simulink model "R7014E_DoubleTankSim2018a"  (R2018a)
settings: Solver=ode5  StartTime=0.0  StopTime=500  RelTol=1e-3  EnableMultiTasking=on
values from neighbouring files (symbols this model uses):
  A = A_const * [-1/sqrt(2*g*(h1+h_eq)) 0 ... (first row only)    [myTank.m]
  B = [6.95/36.2; 0]    [myTank.m]
  C = [0 1]    [myTank.m]
  K = (P*C' + N*R)*inv(R)    [myTank.m]
Description:
  | Double tank process simulation model
  | V1.0
  | 
  | Author: Wolfgang Birk, LTU
settings Model: MinMaxOverflowLogging=ForceOff  Creator=wolfgang  LastModifiedBy=oskwij-4
settings DataIOCC: LimitDataPoints=on  SaveFormat=Array  SignalLoggingSaveFormat=ModelDataLogs
settings OptimizationCC: ExpressionDepthLimit=2147483647  LifeSpan=inf
settings DebuggingCC: UnderspecifiedInitializationDetection=Classic  MergeDetectMultiDrivingBlocksExec=none  SolverPrmCheckMsg=warning  FcnCallInpInsideContextMsg=warning  StateNameClashWarn=warning  SFUnexpectedBacktrackingDiag=warning  SFNoUnconditionalDefaultTransitionDiag=warning  SFExecutionAtInitializationDiag=none
settings HardwareCC: ProdBitPerPointer=32  ProdBitPerSizeT=32  ProdBitPerPtrDiffT=32  ProdLargestAtomicFloat=None  ProdIntDivRoundTo=Undefined  ProdEndianess=Unspecified  ProdWordSize=32  ProdHWDeviceType=32-bit Generic
settings ModelReferenceCC: PropagateSignalLabelsOutOfModel=off
settings CodeAppCC: StateflowObjectComments=on
settings GRTTargetCC: TargetLangStandard=C89/C90 (ANSI)  GeneratePreprocessorConditionals=Disable all
settings ConfigComp: CovMetricSettings=dw  CovHtmlReporting=on  CovSaveCumulativeToWorkspaceVar=on  CovSaveSingleToWorkspaceVar=on  CovExternalEMLEnable=off

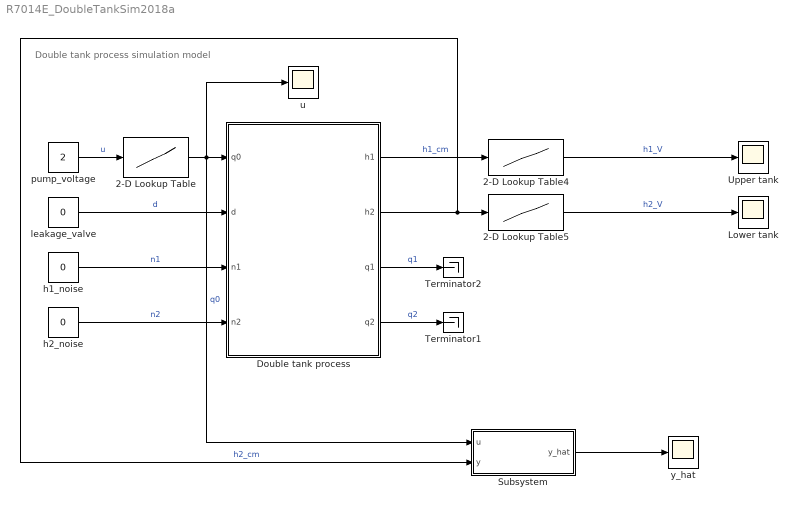
== system R7014E_DoubleTankSim2018a ==
  note: Double tank process simulation model
  2-D Lookup Table : Lookup_n-D  NumberOfTableDimensions=1  BreakpointsForDimension1=x  BreakpointsForDimension2=[1:3]  Table=y  RndMeth=Simplest  InputSameDT=on  mask{x=[0,1,2,3,4,5,6,7,8,9,10], y=|}
      mask y=|
      | [0.0,
      | 0.0,
      | 20.2,
      | 31.9,
      | 40.4,
      | 45.2,
      | 48.7,
      | 52.3,
      | 55.3,
      | 58.5,
      | 63.8]
      mask prompts: x "Values on x-axis"; y "Values on y-axis"
  2-D Lookup Table4 : Lookup_n-D  NumberOfTableDimensions=1  BreakpointsForDimension1=x  BreakpointsForDimension2=[1:3]  Table=y  RndMeth=Simplest  InputSameDT=on  mask{x=[2.50,3.00,3.50,4.00,4.50,5.00,5.50,6.00,6.50,7.00,7.50,8.00,8.50,9.00,9.50,10.00,10.50,11.00,11.50,12.00,12.50,13.00,13.50,14.00,14.50,15.00,15.50], y=[0.21,0.62,1.00,1.49,1.80,2.12,2.54,2.97,3.32,3.71,4.09,4.51,4.87,5.25,5.57,6.04,6.41,6.78,7.13,7.56,7.91,8.32,8.69,9.07,9.42,9.82,9.99]}
      mask prompts: x "Values on x-axis"; y "Values on y-axis"
  2-D Lookup Table5 : Lookup_n-D  NumberOfTableDimensions=1  BreakpointsForDimension1=x  BreakpointsForDimension2=[1:3]  Table=y  RndMeth=Simplest  InputSameDT=on  mask{x=[2.50,3.00,3.50,4.00,4.50,5.00,5.50,6.00,6.50,7.00,7.50,8.00,8.50,9.00,9.50,10.00,10.50,11.00,11.50,12.00,12.50,13.00,13.50,14.00,14.50,15.00,15.50], y=[0.10,0.47,0.87,1.23,1.57,1.98,2.41,2.77,3.16,3.53,3.94,4.32,4.71,5.10,5.46, 5.85, 6.24, 6.63, 7.02, 7.42, 7.74, 8.15, 8.52, 8.90, 9.28, 9.67, 9.94]}
      mask prompts: x "Values on x-axis"; y "Values on y-axis"
  Double tank process : Subsystem  mask{At=33, Ao=0.17, hmax=15.5}
      mask prompts: At "Tank area (cm^2)"; Ao "Opening area (cm^2)"; hmax "Tank height (cm)"
      mask help: Double tank process parameters
  Lower tank : Scope
  Subsystem : Subsystem
  Terminator1 : Terminator
  Terminator2 : Terminator
  Upper tank : Scope
  h1_noise : Constant  Value=0
  h2_noise : Constant  Value=0
  leakage_valve : Constant  Value=0
  pump_voltage : Constant  Value=2
  "u " : Scope
  "y_hat " : Scope
  wires:
  2-D Lookup Table4/1 -> Upper tank/1  "h1_V"
  leakage_valve/1 -> Double tank process/2(d)  "d"
  pump_voltage/1 -> 2-D Lookup Table/1  "u"
  2-D Lookup Table/1 -> Subsystem/1(u), "u "/1, Double tank process/1(q0)  "q0"
  Double tank process/1(h1) -> 2-D Lookup Table4/1  "h1_cm"
  Double tank process/2(h2) -> Subsystem/2(y), 2-D Lookup Table5/1  "h2_cm"
  Double tank process/4(q2) -> Terminator1/1  "q2"
  2-D Lookup Table5/1 -> Lower tank/1  "h2_V"
  Double tank process/3(q1) -> Terminator2/1  "q1"
  h1_noise/1 -> Double tank process/3(n1)  "n1"
  h2_noise/1 -> Double tank process/4(n2)  "n2"
  Subsystem/1("y_hat ") -> "y_hat "/1

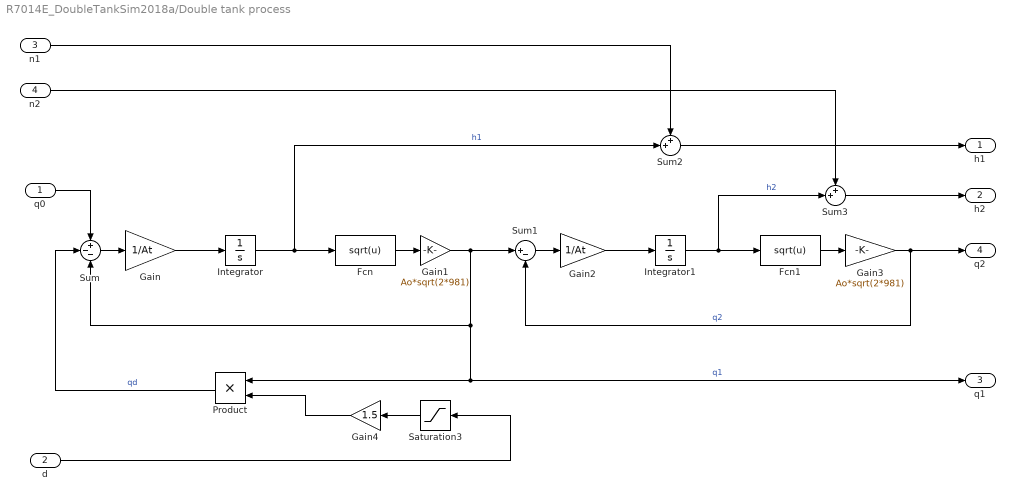
== system R7014E_DoubleTankSim2018a/Double tank process ==
  q0 : Inport
  d : Inport  Port=2
  n1 : Inport  Port=3
  n2 : Inport  Port=4
  Fcn : Fcn  Expr=sqrt(u)
  Fcn1 : Fcn  Expr=sqrt(u)
  Gain : Gain  Gain=1/At
  Gain1 : Gain  Gain=Ao*sqrt(2*981)
  Gain2 : Gain  Gain=1/At
  Gain3 : Gain  Gain=Ao*sqrt(2*981)
  Gain4 : Gain  Gain=1.5
  Integrator : Integrator  LimitOutput=on  UpperSaturationLimit=hmax  LowerSaturationLimit=0
  Integrator1 : Integrator  LimitOutput=on  UpperSaturationLimit=hmax  LowerSaturationLimit=0
  Product : Product  RndMeth=Zero
  Saturation3 : Saturate  UpperLimit=1  LowerLimit=0
  Sum : Sum  Inputs=+--
  Sum1 : Sum  Inputs=|+-
  Sum2 : Sum  Inputs=++|
  Sum3 : Sum  Inputs=++|
  h1 : Outport
  h2 : Outport  Port=2
  q1 : Outport  Port=3
  q2 : Outport  Port=4
  wires:
  Sum/1 -> Gain/1
  Gain/1 -> Integrator/1
  Fcn/1 -> Gain1/1
  Gain1/1 -> Sum1/1, Product/1, q1/1, Sum/3  "q1"
  Sum1/1 -> Gain2/1
  Gain2/1 -> Integrator1/1
  Fcn1/1 -> Gain3/1
  Gain3/1 -> Sum1/2, q2/1  "q2"
  q0/1 -> Sum/1
  Integrator/1 -> Sum2/2, Fcn/1  "h1"
  Product/1 -> Sum/2  "qd"
  d/1 -> Saturation3/1
  Integrator1/1 -> Sum3/2, Fcn1/1  "h2"
  Saturation3/1 -> Gain4/1
  Gain4/1 -> Product/2
  Sum2/1 -> h1/1
  n1/1 -> Sum2/1
  Sum3/1 -> h2/1
  n2/1 -> Sum3/1

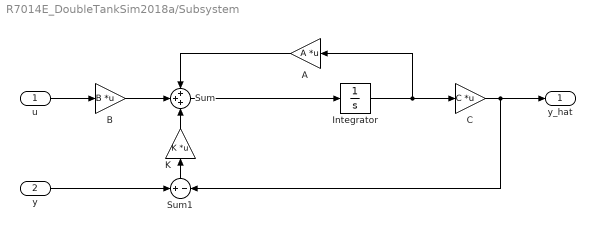
== system R7014E_DoubleTankSim2018a/Subsystem ==
  u : Inport
  y : Inport  Port=2
  A : Gain  Gain=A  Multiplication=Matrix(K*u)
  B : Gain  Gain=B  Multiplication=Matrix(K*u)
  C : Gain  Gain=C  Multiplication=Matrix(K*u)
  Integrator : Integrator
  K : Gain  Gain=K  Multiplication=Matrix(K*u)
  Sum : Sum  Inputs=+++
  Sum1 : Sum  Inputs=+|-
  "y_hat " : Outport
  wires:
  u/1 -> B/1
  Integrator/1 -> C/1, A/1
  Sum/1 -> Integrator/1
  C/1 -> "y_hat "/1, Sum1/2
  y/1 -> Sum1/1
  Sum1/1 -> K/1
  K/1 -> Sum/3
  B/1 -> Sum/2
  A/1 -> Sum/1
